simulink model "Lecture9ICE"  (R2022a)
settings: Solver=VariableStepAuto  StartTime=0.0  StopTime=1800.0  RelTol=1e-3
settings Model: Creator=izacu  LastModifiedBy=izacu

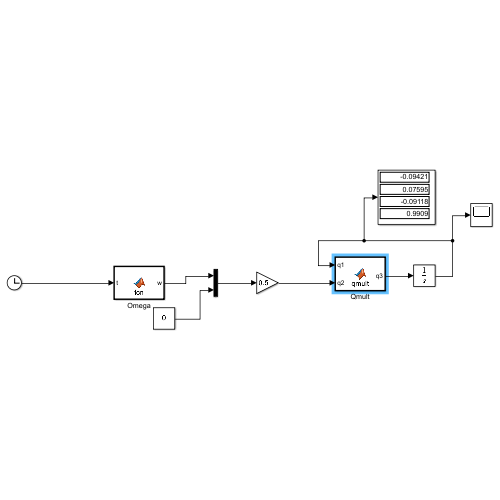
[thumbnail: Simulink's stored preview of the top-level diagram]
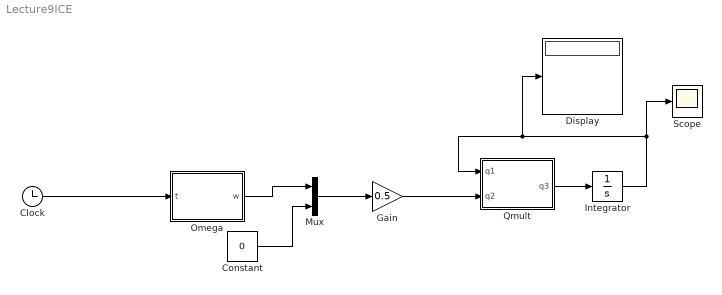
== system Lecture9ICE ==
  Clock : Clock
  Constant : Constant  Value=0
  Display : Display
  Gain : Gain  Gain=0.5
  Integrator : Integrator  InitialCondition=[0;0;0;1]
  Mux : Mux  Inputs=2
  Omega : MATLAB Function  TreatAsAtomicUnit=on
  Qmult : MATLAB Function  TreatAsAtomicUnit=on
  Scope : Scope
  wires:
  Clock/1 -> Omega/1(t)
  Mux/1 -> Gain/1
  Omega/1(w) -> Mux/1
  Constant/1 -> Mux/2
  Gain/1 -> Qmult/2(q2)
  Qmult/1(q3) -> Integrator/1
  Integrator/1 -> Scope/1, Display/1, Qmult/1(q1)

== matlab function Lecture9ICE/Omega ==
  data: t input; w output
function w = fcn(t)

w = 2*pi/300 *[sin(2*pi*t/60);cos(2*pi*t/80);cos(2*pi*t/70)];

== matlab function Lecture9ICE/Qmult ==
  data: q1 input; q3 output; q2 input
function q3 = qmult(q1,q2)

q3 = [q2(4).*q1(1:3) + q1(4).*q2(1:3) - cross(q2(1:3),q1(1:3));
    q2(4)*q1(4) - dot(q2(1:3),q1(1:3))];
